simulink model "model"  (R2018a)
settings: Solver=VariableStepAuto  StartTime=0.0  StopTime=5  RelTol=1e-3
libraries: fuzblock x1, simulink x1
settings Model: Creator=siati  LastModifiedBy=siati

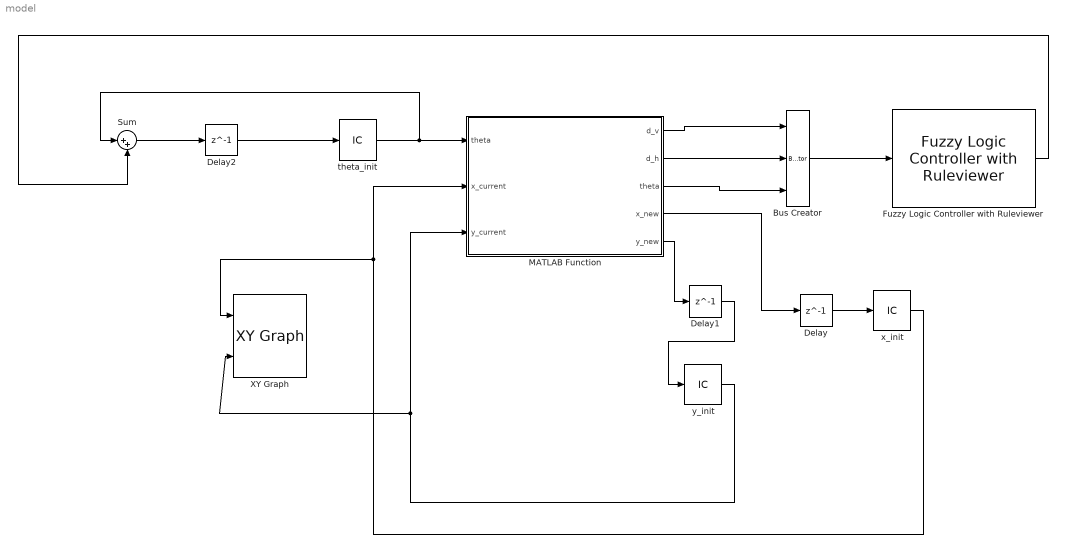
== system model ==
  Bus Creator : BusCreator  Inputs=3
  Delay : Delay  DelayLength=1  InitialCondition=0
  Delay1 : Delay  DelayLength=1  InitialCondition=0
  Delay2 : Delay  DelayLength=1  InitialCondition=0
  Fuzzy Logic Controller with Ruleviewer : fuzblock/Fuzzy Logic  Controller  with Ruleviewer  fismatrix=FLC  Ts=0.01
  MATLAB Function : MATLAB Function  TreatAsAtomicUnit=on
  Sum : Sum  Inputs=|++
  XY Graph : simulink/Sinks/XY Graph  xmin=0  xmax=10  ymin=0  ymax=4  st=-1
  theta_init : InitialCondition  Value=0
  x_init : InitialCondition  Value=4.1
  y_init : InitialCondition  Value=0.3
  wires:
  MATLAB Function/1(d_v) -> Bus Creator/1
  MATLAB Function/2(d_h) -> Bus Creator/2
  MATLAB Function/3(theta) -> Bus Creator/3
  Bus Creator/1 -> Fuzzy Logic Controller with Ruleviewer/1
  MATLAB Function/5(y_new) -> Delay1/1
  MATLAB Function/4(x_new) -> Delay/1
  Delay/1 -> x_init/1
  Delay1/1 -> y_init/1
  Delay2/1 -> theta_init/1
  x_init/1 -> XY Graph/1, MATLAB Function/2(x_current)
  y_init/1 -> XY Graph/2, MATLAB Function/3(y_current)
  theta_init/1 -> Sum/1, MATLAB Function/1("theta ")
  Sum/1 -> Delay2/1
  Fuzzy Logic Controller with Ruleviewer/1 -> Sum/2

== matlab function model/MATLAB Function ==
  data: theta input; d_v output; x_current input; y_current input; d_h output; theta output; x_new output; y_new output
function [d_v, d_h, theta, x_new, y_new] = fcn(theta, x_current, y_current)
    
    %orizw mia voithitiki synarthsh gia ta oria twn metavlhtwn
    
    function f = clamp(k, low, high)
        f = min(max(k, low),high);
    end  
    
    %h theta prepei na anhkei sto [-180,180]
    
    theta = clamp(theta, -180, 180);
    
    %metatrepw th gwnia se rads kai orizw thn taxythta tou oxhmatos

    theta_rads = (2*pi*theta)/360;
    
    if (x_current == 10)
        
        u = 0;
        
    else
        
        u = 0.05;
        
    end  
    
    %ypologizw th metatopish
    
    dx = u*cos(theta_rads);
    dy = u*sin(theta_rads);
    
    %ypologizw th nea thesh tou oxhmatos
    
    x_new = x_current + dx;
    y_new = y_current + dy;
    
    %ypologizw to dv
    
    if(x_new < 5)
        d_v = y_new;
    elseif(x_new < 6)
        d_v = y_new - 1;
    elseif(x_new < 7)
        d_v = y_new - 2;
    else
        d_v = y_new - 3;
    end
    
    %ypologizw to dh
    
    if(y_new < 1)
        d_h = 5 - x_new;
    elseif(y_new < 2)
        d_h = 6 - x_new;
    elseif(y_new < 3)
        d_h = 7 - x_new;
    else
        d_h = 1;
    end
    
    %to dv kai to dh prepei na anhkoun sto [0,1]
    
    d_v = clamp(d_v, 0, 1);
    d_h = clamp(d_h, 0, 1);
    
end
